simulink model "White_Activity9_sim"  (R2020b)
settings: Solver=VariableStepAuto  StartTime=0.0  StopTime=10.0  RelTol=1e-3
values from neighbouring files (symbols this model uses):
  m = 4    [White_Activity9.m]
settings Model: Creator=Michael  LastModifiedBy=Michael
settings OptimizationCC: BlockReduction=off  DefaultParameterBehavior=Inlined  BufferReuse=off

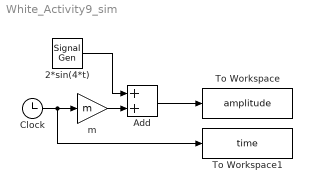
== system White_Activity9_sim ==
  2*sin(4*t) : SignalGenerator  Amplitude=2  Frequency=4  Units=rad/sec
  Add : Sum
  Clock : Clock
  To Workspace : ToWorkspace  VariableName=amplitude  SampleTime=-1
  To Workspace1 : ToWorkspace  VariableName=time  SampleTime=-1
  m : Gain  Gain=m
  wires:
  Clock/1 -> To Workspace1/1, m/1
  m/1 -> Add/2
  2*sin(4*t)/1 -> Add/1
  Add/1 -> To Workspace/1
